simulink model "Q_learning_rotor_v3_min_M_imp"  (R2021a)
settings: Solver=VariableStepAuto  StartTime=0.0  StopTime=Tf  RelTol=1e-3
values from neighbouring files (symbols this model uses):
  Ator = pi*r^2    (= 0.00125663706144)    [INIT_rotor.m]    (also in rotor_DataFile.m)
  bd = 20    [INIT_rotor.m]    (also in rotor_DataFile.m)
  deltam = 0    [INIT_rotor.m]    (also in rotor_DataFile.m = 3e-05)
  dumax = ustavka+0.2e-3    (= 0.0034)    [INIT_Q_rotor.m]
  dumin = ustavka-0.2e-3    (= 0.003)    [INIT_Q_rotor.m]
  kd = 8e3    (= 8000)    [INIT_rotor.m]    (also in rotor_DataFile.m)
  Kr = 1000    [INIT_Q_rotor.m]
  n = -3e+3    (= -3000)    [INIT_rotor.m]    (also in rotor_DataFile.m)
  p0 = 1.08e5    (= 108000)    [rotor_DataFile.m]
  p00 = 1.05e5    (= 105000)    [rotor_DataFile.m]
  p0max = 1.1e5    (= 110000)    [INIT_Q_rotor.m]
  p0min = 1.05e5    (= 105000)    [INIT_Q_rotor.m]
  p1 = 1.08e5    (= 108000)    [rotor_DataFile.m]
  p10 = 1.00e5    (= 100000)    [rotor_DataFile.m]
  p11 = 1.00e5    (= 100000)    [INIT_rotor.m]
  p1max = 1.08e5    (= 108000)    [INIT_Q_rotor.m]
  p1min = 1e5    (= 100000)    [INIT_Q_rotor.m]
  Tf = 4    [INIT_Q_rotor.m]
  ustavka = 3.2e-3    (= 0.0032)    [INIT_Q_rotor.m]
  X10 = 1    [INIT_rotor.m]    (also in rotor_DataFile.m = 0)
  X20 = 0    [INIT_rotor.m]    (also in rotor_DataFile.m)
  X30 = 200    [INIT_rotor.m]
undefined symbols (not defined in the file or in its folder): smiData, X, Y, Z
libraries: neural x80, sm_lib x21, nesl_utility x14, simulink x7, dspmathops x3, pid_lib x1, rllib x1
(part 4 of 4)

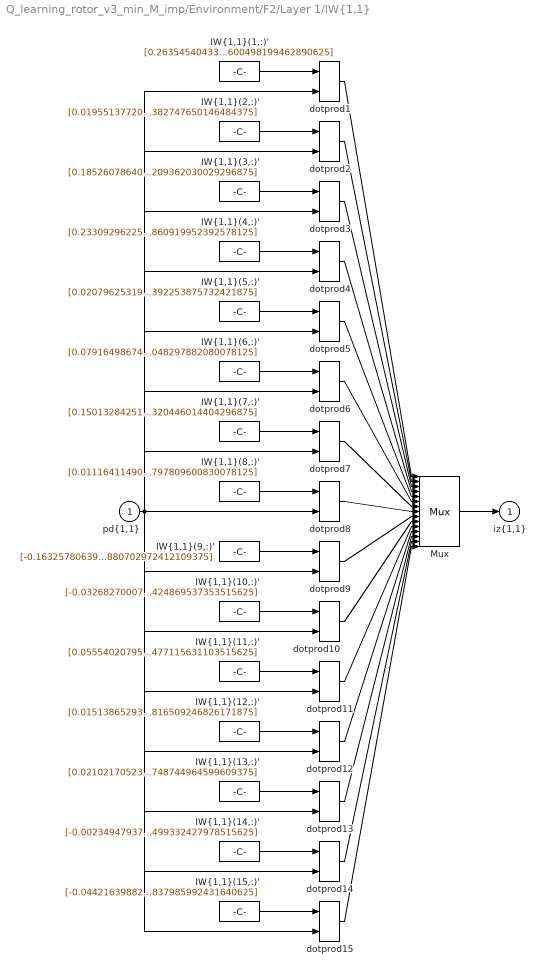
== system Q_learning_rotor_v3_min_M_imp/Environment/F2/Layer 1/IW{1,1} ==
  "pd{1,1}" : Inport  PortDimensions=8
      mask Display: e = 0.06;c1 = [120 230 180]/255;c2 = ([120 230 180]+0)/(256+128);c3 = ([120 230 180]+128)/(256+128);patch([0 1 1 0],[0 0 1 1],c1);patch([0 1 1 1-e 1-e 0+e],[0 0 1 1-e 0+e 0+e],c2);patch([0 0 1 1-e 0+e 0+e],[0 1 1 1-e 1-e 0+e],c3);plot([0 1 1 0 0],[0 0 1 1 0]);
  "IW{1,1}(1,:)'" : Constant  Value=[0.263545404332929056323564509511925280094146728515625;0.0280744574899199593465137780867735273204743862152099609375;0.785332970886842840485542183159850537776947021484375;-2.400750927396896106102985868346877396106719970703125;-1.03350617396331045938495662994682788848876953125;-1.2258655255748223122935769424657337367534637451171875;0.1567087824745667379300329002944636158645153045654296875;0.1216734266486191595735277815037989057600498199462890625]
      mask Display: e = 0.06;c1 = [120 150 230]/255;c2 = ([120 150 230]+0)/383;c3 = ([120 150 230]+128)/383;patch([0 1 1 0],[0 0 1 1],c1);patch([0 1 1 1-e 1-e 0+e],[0 0 1 1-e 0+e 0+e],c2);patch([0 0 1 1-e 0+e 0+e],[0 1 1 1-e 1-e 0+e],c3);plot([0 1 1 0 0],[0 0 1 1 0]);disp('Weights');
  "IW{1,1}(10,:)'" : Constant  Value=[-0.032682700078258054843249880150324315764009952545166015625;0.03781420832800962139597089617382152937352657318115234375;-1.3144429617808779386933792920899577438831329345703125;-2.681476711076717034387684179819189012050628662109375;-1.9744435884615196830083050372195430099964141845703125;0.94119793184532640761830180053948424756526947021484375;-1.019077215252574664106077761971391737461090087890625;0.0192143505873720345233923723071711719967424869537353515625]
      mask Display: e = 0.06;c1 = [120 150 230]/255;c2 = ([120 150 230]+0)/383;c3 = ([120 150 230]+128)/383;patch([0 1 1 0],[0 0 1 1],c1);patch([0 1 1 1-e 1-e 0+e],[0 0 1 1-e 0+e 0+e],c2);patch([0 0 1 1-e 0+e 0+e],[0 1 1 1-e 1-e 0+e],c3);plot([0 1 1 0 0],[0 0 1 1 0]);disp('Weights');
  "IW{1,1}(11,:)'" : Constant  Value=[0.055540207952238344890627530503479647450149059295654296875;0.00866395649697577173442564202332505374215543270111083984375;-0.1495569984123192586178419105635839514434337615966796875;-1.2041741748349570340081982067204080522060394287109375;-0.56109907977361472841693057489464990794658660888671875;-0.367585963305995855332497512790723703801631927490234375;-0.4099183908587580305038500227965414524078369140625;0.032207486974964817660893601214411319233477115631103515625]
      mask Display: e = 0.06;c1 = [120 150 230]/255;c2 = ([120 150 230]+0)/383;c3 = ([120 150 230]+128)/383;patch([0 1 1 0],[0 0 1 1],c1);patch([0 1 1 1-e 1-e 0+e],[0 0 1 1-e 0+e 0+e],c2);patch([0 0 1 1-e 0+e 0+e],[0 1 1 1-e 1-e 0+e],c3);plot([0 1 1 0 0],[0 0 1 1 0]);disp('Weights');
  "IW{1,1}(12,:)'" : Constant  Value=[0.01513865293832539204998965942650102078914642333984375;-0.007286743139548861221410636090922707808203995227813720703125;0.08408901881263618205419874129802337847650051116943359375;0.14107413188811068760486477913218550384044647216796875;1.2293671603681011195163819138542748987674713134765625;0.405997235974045300732626628814614377915859222412109375;-0.93506324769651960604477380911703221499919891357421875;-0.00684806045102126330348379923407264868728816509246826171875]
      mask Display: e = 0.06;c1 = [120 150 230]/255;c2 = ([120 150 230]+0)/383;c3 = ([120 150 230]+128)/383;patch([0 1 1 0],[0 0 1 1],c1);patch([0 1 1 1-e 1-e 0+e],[0 0 1 1-e 0+e 0+e],c2);patch([0 0 1 1-e 0+e 0+e],[0 1 1 1-e 1-e 0+e],c3);plot([0 1 1 0 0],[0 0 1 1 0]);disp('Weights');
  "IW{1,1}(13,:)'" : Constant  Value=[0.0210217052303556528602968000996042974293231964111328125;-0.032273386069569386103150776534675969742238521575927734375;0.1523531376308588647372488367182086221873760223388671875;-0.50578406248212903761896086507476866245269775390625;-1.2148553203552625578964807573356665670871734619140625;0.93089507593940756802197711294866167008876800537109375;0.8797008886075923239644680506899021565914154052734375;-0.01011072435612333196564005532991359359584748744964599609375]
      mask Display: e = 0.06;c1 = [120 150 230]/255;c2 = ([120 150 230]+0)/383;c3 = ([120 150 230]+128)/383;patch([0 1 1 0],[0 0 1 1],c1);patch([0 1 1 1-e 1-e 0+e],[0 0 1 1-e 0+e 0+e],c2);patch([0 0 1 1-e 0+e 0+e],[0 1 1 1-e 1-e 0+e],c3);plot([0 1 1 0 0],[0 0 1 1 0]);disp('Weights');
  "IW{1,1}(14,:)'" : Constant  Value=[-0.002349479374296047085035610280101536773145198822021484375;-0.015503507698309160200977885324391536414623260498046875;-0.393141378679239650306698194981436245143413543701171875;0.10230100857625297472441872059789602644741535186767578125;-0.0985401080283706265472432050955831073224544525146484375;0.256601592956030966075076094057294540107250213623046875;-0.69141570456732670546529107014066539704799652099609375;0.061357359811551694106501741998727084137499332427978515625]
      mask Display: e = 0.06;c1 = [120 150 230]/255;c2 = ([120 150 230]+0)/383;c3 = ([120 150 230]+128)/383;patch([0 1 1 0],[0 0 1 1],c1);patch([0 1 1 1-e 1-e 0+e],[0 0 1 1-e 0+e 0+e],c2);patch([0 0 1 1-e 0+e 0+e],[0 1 1 1-e 1-e 0+e],c3);plot([0 1 1 0 0],[0 0 1 1 0]);disp('Weights');
  "IW{1,1}(15,:)'" : Constant  Value=[-0.044216398821182827105769064246487687341868877410888671875;0.0150412139294658873944765531405209912918508052825927734375;-0.56415725694198382011990133833023719489574432373046875;1.5027241430763869090014850371517241001129150390625;0.355737529627508541896219185218797065317630767822265625;0.67099091817371192547625469160266220569610595703125;0.864116878011450761931655506487004458904266357421875;-0.07105011406486406999594152011923142708837985992431640625]
      mask Display: e = 0.06;c1 = [120 150 230]/255;c2 = ([120 150 230]+0)/383;c3 = ([120 150 230]+128)/383;patch([0 1 1 0],[0 0 1 1],c1);patch([0 1 1 1-e 1-e 0+e],[0 0 1 1-e 0+e 0+e],c2);patch([0 0 1 1-e 0+e 0+e],[0 1 1 1-e 1-e 0+e],c3);plot([0 1 1 0 0],[0 0 1 1 0]);disp('Weights');
  "IW{1,1}(2,:)'" : Constant  Value=[0.0195513772009782982319592292697052471339702606201171875;-0.01018554910181642715605310200999156222678720951080322265625;1.0376137849348501251967036296264268457889556884765625;0.403408290930529156437245319466455839574337005615234375;-0.665510220609730307472773347399197518825531005859375;-0.51058035967489578954570106361643411219120025634765625;1.0007272117893375451558313216082751750946044921875;0.019596135259655055038674476008964120410382747650146484375]
      mask Display: e = 0.06;c1 = [120 150 230]/255;c2 = ([120 150 230]+0)/383;c3 = ([120 150 230]+128)/383;patch([0 1 1 0],[0 0 1 1],c1);patch([0 1 1 1-e 1-e 0+e],[0 0 1 1-e 0+e 0+e],c2);patch([0 0 1 1-e 0+e 0+e],[0 1 1 1-e 1-e 0+e],c3);plot([0 1 1 0 0],[0 0 1 1 0]);disp('Weights');
  "IW{1,1}(3,:)'" : Constant  Value=[0.1852607864006721449801062817641650326550006866455078125;-0.035421893108780903858257005367704550735652446746826171875;-0.96238883016556642235883600733359344303607940673828125;-0.1398795408219530578275424659295822493731975555419921875;0.043315733871104648844418960607072222046554088592529296875;0.74905077928134866649401146787567995488643646240234375;-1.3480146194933546599514784247730858623981475830078125;0.158637073539034278990556003918754868209362030029296875]
      mask Display: e = 0.06;c1 = [120 150 230]/255;c2 = ([120 150 230]+0)/383;c3 = ([120 150 230]+128)/383;patch([0 1 1 0],[0 0 1 1],c1);patch([0 1 1 1-e 1-e 0+e],[0 0 1 1-e 0+e 0+e],c2);patch([0 0 1 1-e 0+e 0+e],[0 1 1 1-e 1-e 0+e],c3);plot([0 1 1 0 0],[0 0 1 1 0]);disp('Weights');
  "IW{1,1}(4,:)'" : Constant  Value=[0.23309296225073039554587239763350225985050201416015625;0.03210029035712336220598217551014386117458343505859375;0.65784775936412243080297912456444464623928070068359375;-2.453647203103570095805707751424051821231842041015625;-1.1857418175884053557211927909520454704761505126953125;-1.0833997280227725124035487169749103486537933349609375;0.053272902877193495374541498676990158855915069580078125;0.12026706771248170391164222792212967760860919952392578125]
      mask Display: e = 0.06;c1 = [120 150 230]/255;c2 = ([120 150 230]+0)/383;c3 = ([120 150 230]+128)/383;patch([0 1 1 0],[0 0 1 1],c1);patch([0 1 1 1-e 1-e 0+e],[0 0 1 1-e 0+e 0+e],c2);patch([0 0 1 1-e 0+e 0+e],[0 1 1 1-e 1-e 0+e],c3);plot([0 1 1 0 0],[0 0 1 1 0]);disp('Weights');
  "IW{1,1}(5,:)'" : Constant  Value=[0.0207962531983513047861844569297318230383098125457763671875;0.0258380085905217903030628434635218582116067409515380859375;-0.75225209845463492097650259893271140754222869873046875;-1.8055881558413087173420308317872695624828338623046875;-1.2661925975772041486067109872237779200077056884765625;0.30820038911983738127986498511745594441890716552734375;-0.69762588488066878955606853196513839066028594970703125;0.043450823381268655065667871895129792392253875732421875]
      mask Display: e = 0.06;c1 = [120 150 230]/255;c2 = ([120 150 230]+0)/383;c3 = ([120 150 230]+128)/383;patch([0 1 1 0],[0 0 1 1],c1);patch([0 1 1 1-e 1-e 0+e],[0 0 1 1-e 0+e 0+e],c2);patch([0 0 1 1-e 0+e 0+e],[0 1 1 1-e 1-e 0+e],c3);plot([0 1 1 0 0],[0 0 1 1 0]);disp('Weights');
  "IW{1,1}(6,:)'" : Constant  Value=[0.0791649867434642551256018805361236445605754852294921875;-0.0208260864341522251852456548704140004701912403106689453125;-0.541038515794388441548790069646202027797698974609375;0.01404869201285276723856210168150937533937394618988037109375;-0.05333402617709774584664472740769269876182079315185546875;0.4645797256487174120564986878889612853527069091796875;-0.86253689600163496731255463600973598659038543701171875;0.08261879415788993263891626384065602906048297882080078125]
      mask Display: e = 0.06;c1 = [120 150 230]/255;c2 = ([120 150 230]+0)/383;c3 = ([120 150 230]+128)/383;patch([0 1 1 0],[0 0 1 1],c1);patch([0 1 1 1-e 1-e 0+e],[0 0 1 1-e 0+e 0+e],c2);patch([0 0 1 1-e 0+e 0+e],[0 1 1 1-e 1-e 0+e],c3);plot([0 1 1 0 0],[0 0 1 1 0]);disp('Weights');
  "IW{1,1}(7,:)'" : Constant  Value=[0.1501328425117599840721283044331357814371585845947265625;-0.1419145374554392213806153222321881912648677825927734375;-0.50031355222014750605552535489550791680812835693359375;1.0439359379314641085301218481617979705333709716796875;0.2296139652304131362203776234309771098196506500244140625;-0.768687381273901682021687520318664610385894775390625;0.327858303858620081516761501916334964334964752197265625;-0.5721788946593224789438636435079388320446014404296875]
      mask Display: e = 0.06;c1 = [120 150 230]/255;c2 = ([120 150 230]+0)/383;c3 = ([120 150 230]+128)/383;patch([0 1 1 0],[0 0 1 1],c1);patch([0 1 1 1-e 1-e 0+e],[0 0 1 1-e 0+e 0+e],c2);patch([0 0 1 1-e 0+e 0+e],[0 1 1 1-e 1-e 0+e],c3);plot([0 1 1 0 0],[0 0 1 1 0]);disp('Weights');
  "IW{1,1}(8,:)'" : Constant  Value=[0.0111641149092882967230888624499129946343600749969482421875;0.019322299447494285795645652115126722492277622222900390625;0.6476794046053793163508771613123826682567596435546875;-1.9590535910084947435194635545485652983188629150390625;-0.95194517339799744615191912089358083903789520263671875;-0.2051910504571095306136641056582448072731494903564453125;-0.34028428786666464755938932285062037408351898193359375;0.1531810528174038232851472685069893486797809600830078125]
      mask Display: e = 0.06;c1 = [120 150 230]/255;c2 = ([120 150 230]+0)/383;c3 = ([120 150 230]+128)/383;patch([0 1 1 0],[0 0 1 1],c1);patch([0 1 1 1-e 1-e 0+e],[0 0 1 1-e 0+e 0+e],c2);patch([0 0 1 1-e 0+e 0+e],[0 1 1 1-e 1-e 0+e],c3);plot([0 1 1 0 0],[0 0 1 1 0]);disp('Weights');
  "IW{1,1}(9,:)'" : Constant  Value=[-0.1632578063934266576762155409596743993461132049560546875;0.049121285080663816546842070920320111326873302459716796875;0.70710307107203906884507205177214927971363067626953125;0.74083810589253185074909424656652845442295074462890625;-0.79287321140284994225311265836353413760662078857421875;0.6505880433479329649770761534455232322216033935546875;0.86903557929343555610302018976653926074504852294921875;-0.17748956420124917254810270605958066880702972412109375]
      mask Display: e = 0.06;c1 = [120 150 230]/255;c2 = ([120 150 230]+0)/383;c3 = ([120 150 230]+128)/383;patch([0 1 1 0],[0 0 1 1],c1);patch([0 1 1 1-e 1-e 0+e],[0 0 1 1-e 0+e 0+e],c2);patch([0 0 1 1-e 0+e 0+e],[0 1 1 1-e 1-e 0+e],c3);plot([0 1 1 0 0],[0 0 1 1 0]);disp('Weights');
  Mux : Mux  Inputs=15
      mask Display: e = 0.06;c1 = [120 150 230]/255;c2 = ([120 150 230]+0)/383;c3 = ([120 150 230]+128)/383;patch([0 1 1 0],[0 0 1 1],c1);patch([0 1 1 1-e 1-e 0+e],[0 0 1 1-e 0+e 0+e],c2);patch([0 0 1 1-e 0+e 0+e],[0 1 1 1-e 1-e 0+e],c3);plot([0 1 1 0 0],[0 0 1 1 0]);disp('Mux');
  dotprod{1..15} (15 alike) : neural/Weight Functions/dotprod
  "iz{1,1}" : Outport
      mask Display: e = 0.06;c1 = [120 230 180]/255;c2 = ([120 230 180]+0)/(256+128);c3 = ([120 230 180]+128)/(256+128);patch([0 1 1 0],[0 0 1 1],c1);patch([0 1 1 1-e 1-e 0+e],[0 0 1 1-e 0+e 0+e],c2);patch([0 0 1 1-e 0+e 0+e],[0 1 1 1-e 1-e 0+e],c3);plot([0 1 1 0 0],[0 0 1 1 0]);
  wires:
  "IW{1,1}(1,:)'"/1 -> dotprod1/1
  "pd{1,1}"/1 -> dotprod1/2, dotprod2/2, dotprod3/2, dotprod4/2, dotprod5/2, dotprod6/2, dotprod7/2, dotprod8/2, dotprod9/2, dotprod10/2, dotprod11/2, dotprod12/2, dotprod13/2, dotprod14/2, dotprod15/2
  dotprod1/1 -> Mux/1
  "IW{1,1}(2,:)'"/1 -> dotprod2/1
  dotprod2/1 -> Mux/2
  "IW{1,1}(3,:)'"/1 -> dotprod3/1
  dotprod3/1 -> Mux/3
  "IW{1,1}(4,:)'"/1 -> dotprod4/1
  dotprod4/1 -> Mux/4
  "IW{1,1}(5,:)'"/1 -> dotprod5/1
  dotprod5/1 -> Mux/5
  "IW{1,1}(6,:)'"/1 -> dotprod6/1
  dotprod6/1 -> Mux/6
  "IW{1,1}(7,:)'"/1 -> dotprod7/1
  dotprod7/1 -> Mux/7
  "IW{1,1}(8,:)'"/1 -> dotprod8/1
  dotprod8/1 -> Mux/8
  "IW{1,1}(9,:)'"/1 -> dotprod9/1
  dotprod9/1 -> Mux/9
  "IW{1,1}(10,:)'"/1 -> dotprod10/1
  dotprod10/1 -> Mux/10
  "IW{1,1}(11,:)'"/1 -> dotprod11/1
  dotprod11/1 -> Mux/11
  "IW{1,1}(12,:)'"/1 -> dotprod12/1
  dotprod12/1 -> Mux/12
  "IW{1,1}(13,:)'"/1 -> dotprod13/1
  dotprod13/1 -> Mux/13
  "IW{1,1}(14,:)'"/1 -> dotprod14/1
  dotprod14/1 -> Mux/14
  "IW{1,1}(15,:)'"/1 -> dotprod15/1
  dotprod15/1 -> Mux/15
  Mux/1 -> "iz{1,1}"/1

== system Q_learning_rotor_v3_min_M_imp/Environment/F2/Layer 2/Delays 1 ==
  "p{2}" : Inport  PortDimensions=15
      mask Display: e = 0.06;c1 = [120 230 180]/255;c2 = ([120 230 180]+0)/(256+128);c3 = ([120 230 180]+128)/(256+128);patch([0 1 1 0],[0 0 1 1],c1);patch([0 1 1 1-e 1-e 0+e],[0 0 1 1-e 0+e 0+e],c2);patch([0 0 1 1-e 0+e 0+e],[0 1 1 1-e 1-e 0+e],c3);plot([0 1 1 0 0],[0 0 1 1 0]);
  mux : Mux  Inputs=1
      mask Display: e = 0.06;c1 = [120 150 230]/255;c2 = ([120 150 230]+0)/383;c3 = ([120 150 230]+128)/383;patch([0 1 1 0],[0 0 1 1],c1);patch([0 1 1 1-e 1-e 0+e],[0 0 1 1-e 0+e 0+e],c2);patch([0 0 1 1-e 0+e 0+e],[0 1 1 1-e 1-e 0+e],c3);plot([0 1 1 0 0],[0 0 1 1 0]);disp('Mux')
  "pd{2,1}" : Outport
      mask Display: e = 0.06;c1 = [120 230 180]/255;c2 = ([120 230 180]+0)/(256+128);c3 = ([120 230 180]+128)/(256+128);patch([0 1 1 0],[0 0 1 1],c1);patch([0 1 1 1-e 1-e 0+e],[0 0 1 1-e 0+e 0+e],c2);patch([0 0 1 1-e 0+e 0+e],[0 1 1 1-e 1-e 0+e],c3);plot([0 1 1 0 0],[0 0 1 1 0]);
  wires:
  "p{2}"/1 -> mux/1
  mux/1 -> "pd{2,1}"/1

== system Q_learning_rotor_v3_min_M_imp/Environment/F2/Layer 2/LW{2,1} ==
  "ad{2,1}" : Inport  PortDimensions=15
      mask Display: e = 0.06;c1 = [120 230 180]/255;c2 = ([120 230 180]+0)/(256+128);c3 = ([120 230 180]+128)/(256+128);patch([0 1 1 0],[0 0 1 1],c1);patch([0 1 1 1-e 1-e 0+e],[0 0 1 1-e 0+e 0+e],c2);patch([0 0 1 1-e 0+e 0+e],[0 1 1 1-e 1-e 0+e],c3);plot([0 1 1 0 0],[0 0 1 1 0]);
  "IW{2,1}(1,:)'" : Constant  Value=[-2.8839445060521295971511790412478148937225341796875;7.68490157682992514054376442800275981426239013671875;1.6083510919674959271929992610239423811435699462890625;3.49943182265510532857888392754830420017242431640625;-3.8525253166788360204009222798049449920654296875;-5.88610951123064385370753370807506144046783447265625;0.033877648943551226523585029326568474061787128448486328125;-3.281568649392260450525782289332710206508636474609375;0.2124320347898714100853823083525639958679676055908203125;1.26767619245783347281530950567685067653656005859375;1.6439680904654132564957080830936320126056671142578125;-3.4066905868457890704803503467701375484466552734375;-9.6163191123424436312916441238485276699066162109375;4.4120135957978714458249669405631721019744873046875;-4.388737037437319798982571228407323360443115234375]
      mask Display: e = 0.06;c1 = [120 150 230]/255;c2 = ([120 150 230]+0)/383;c3 = ([120 150 230]+128)/383;patch([0 1 1 0],[0 0 1 1],c1);patch([0 1 1 1-e 1-e 0+e],[0 0 1 1-e 0+e 0+e],c2);patch([0 0 1 1-e 0+e 0+e],[0 1 1 1-e 1-e 0+e],c3);plot([0 1 1 0 0],[0 0 1 1 0]);disp('weights');
  Mux : Mux  Inputs=1
      mask Display: e = 0.06;c1 = [120 150 230]/255;c2 = ([120 150 230]+0)/383;c3 = ([120 150 230]+128)/383;patch([0 1 1 0],[0 0 1 1],c1);patch([0 1 1 1-e 1-e 0+e],[0 0 1 1-e 0+e 0+e],c2);patch([0 0 1 1-e 0+e 0+e],[0 1 1 1-e 1-e 0+e],c3);plot([0 1 1 0 0],[0 0 1 1 0]);disp('Mux');
  dotprod1 : neural/Weight Functions/dotprod
  "lz{2,1}" : Outport
      mask Display: e = 0.06;c1 = [120 230 180]/255;c2 = ([120 230 180]+0)/(256+128);c3 = ([120 230 180]+128)/(256+128);patch([0 1 1 0],[0 0 1 1],c1);patch([0 1 1 1-e 1-e 0+e],[0 0 1 1-e 0+e 0+e],c2);patch([0 0 1 1-e 0+e 0+e],[0 1 1 1-e 1-e 0+e],c3);plot([0 1 1 0 0],[0 0 1 1 0]);
  wires:
  "IW{2,1}(1,:)'"/1 -> dotprod1/1
  "ad{2,1}"/1 -> dotprod1/2
  dotprod1/1 -> Mux/1
  Mux/1 -> "lz{2,1}"/1

== system Q_learning_rotor_v3_min_M_imp/Environment/F3/Layer 1/Delays 1 ==
  "p{1}" : Inport  PortDimensions=8
      mask Display: e = 0.06;c1 = [120 230 180]/255;c2 = ([120 230 180]+0)/(256+128);c3 = ([120 230 180]+128)/(256+128);patch([0 1 1 0],[0 0 1 1],c1);patch([0 1 1 1-e 1-e 0+e],[0 0 1 1-e 0+e 0+e],c2);patch([0 0 1 1-e 0+e 0+e],[0 1 1 1-e 1-e 0+e],c3);plot([0 1 1 0 0],[0 0 1 1 0]);
  mux : Mux  Inputs=1
      mask Display: e = 0.06;c1 = [120 150 230]/255;c2 = ([120 150 230]+0)/383;c3 = ([120 150 230]+128)/383;patch([0 1 1 0],[0 0 1 1],c1);patch([0 1 1 1-e 1-e 0+e],[0 0 1 1-e 0+e 0+e],c2);patch([0 0 1 1-e 0+e 0+e],[0 1 1 1-e 1-e 0+e],c3);plot([0 1 1 0 0],[0 0 1 1 0]);disp('Mux')
  "pd{1,1}" : Outport
      mask Display: e = 0.06;c1 = [120 230 180]/255;c2 = ([120 230 180]+0)/(256+128);c3 = ([120 230 180]+128)/(256+128);patch([0 1 1 0],[0 0 1 1],c1);patch([0 1 1 1-e 1-e 0+e],[0 0 1 1-e 0+e 0+e],c2);patch([0 0 1 1-e 0+e 0+e],[0 1 1 1-e 1-e 0+e],c3);plot([0 1 1 0 0],[0 0 1 1 0]);
  wires:
  "p{1}"/1 -> mux/1
  mux/1 -> "pd{1,1}"/1

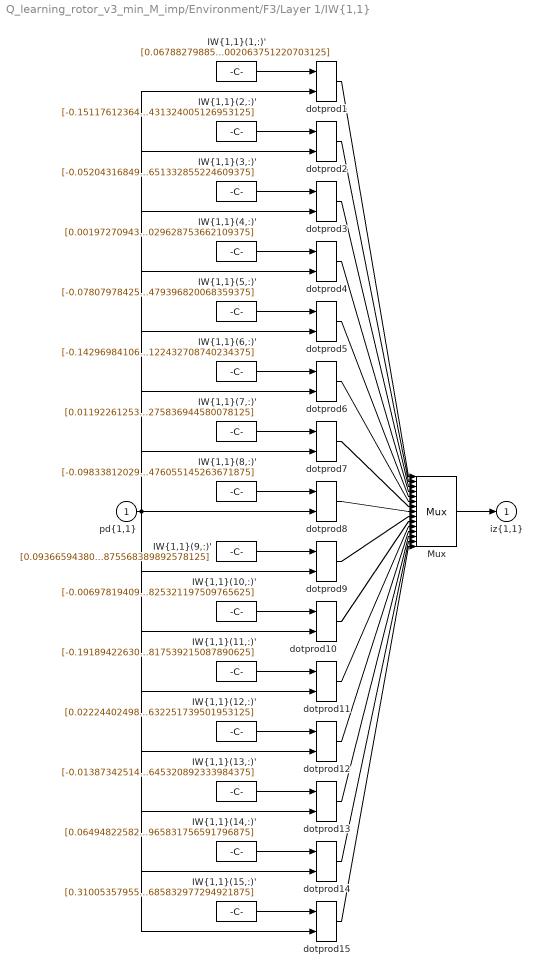
== system Q_learning_rotor_v3_min_M_imp/Environment/F3/Layer 1/IW{1,1} ==
  "pd{1,1}" : Inport  PortDimensions=8
      mask Display: e = 0.06;c1 = [120 230 180]/255;c2 = ([120 230 180]+0)/(256+128);c3 = ([120 230 180]+128)/(256+128);patch([0 1 1 0],[0 0 1 1],c1);patch([0 1 1 1-e 1-e 0+e],[0 0 1 1-e 0+e 0+e],c2);patch([0 0 1 1-e 0+e 0+e],[0 1 1 1-e 1-e 0+e],c3);plot([0 1 1 0 0],[0 0 1 1 0]);
  "IW{1,1}(1,:)'" : Constant  Value=[0.06788279885655380818665349806906306184828281402587890625;-0.00992236614156143115206276661410811357200145721435546875;0.128807470069277008040131704547093249857425689697265625;-2.07557374820626261424649783293716609477996826171875;-1.3371842639701483346215127312461845576763153076171875;-2.173773926338138817726530760410241782665252685546875;-0.854299781709458638800924745737574994564056396484375;0.06477886523293803489043085619414341636002063751220703125]
      mask Display: e = 0.06;c1 = [120 150 230]/255;c2 = ([120 150 230]+0)/383;c3 = ([120 150 230]+128)/383;patch([0 1 1 0],[0 0 1 1],c1);patch([0 1 1 1-e 1-e 0+e],[0 0 1 1-e 0+e 0+e],c2);patch([0 0 1 1-e 0+e 0+e],[0 1 1 1-e 1-e 0+e],c3);plot([0 1 1 0 0],[0 0 1 1 0]);disp('Weights');
  "IW{1,1}(10,:)'" : Constant  Value=[-0.006978194095090421711358175116401980631053447723388671875;0.00922221332153015660448858170639141462743282318115234375;-0.330894108761513872085657794741564430296421051025390625;0.8886342899794936744939377604168839752674102783203125;-0.351152275670796931716921562838251702487468719482421875;0.9474812931835525642298989623668603599071502685546875;1.021305796765827000882609354448504745960235595703125;-0.037725419671657024756061815651264623738825321197509765625]
      mask Display: e = 0.06;c1 = [120 150 230]/255;c2 = ([120 150 230]+0)/383;c3 = ([120 150 230]+128)/383;patch([0 1 1 0],[0 0 1 1],c1);patch([0 1 1 1-e 1-e 0+e],[0 0 1 1-e 0+e 0+e],c2);patch([0 0 1 1-e 0+e 0+e],[0 1 1 1-e 1-e 0+e],c3);plot([0 1 1 0 0],[0 0 1 1 0]);disp('Weights');
  "IW{1,1}(11,:)'" : Constant  Value=[-0.1918942263094554900870747360386303626000881195068359375;-0.0045254450572274999842203868638534913770854473114013671875;0.898112362451640944271957778255455195903778076171875;0.216610886716492812009704493902972899377346038818359375;-0.5903638625466645084571837287512607872486114501953125;-2.03988383709788489994707560981623828411102294921875;0.133448489177298179608754935543402098119258880615234375;0.149400957588209204462970092208706773817539215087890625]
      mask Display: e = 0.06;c1 = [120 150 230]/255;c2 = ([120 150 230]+0)/383;c3 = ([120 150 230]+128)/383;patch([0 1 1 0],[0 0 1 1],c1);patch([0 1 1 1-e 1-e 0+e],[0 0 1 1-e 0+e 0+e],c2);patch([0 0 1 1-e 0+e 0+e],[0 1 1 1-e 1-e 0+e],c3);plot([0 1 1 0 0],[0 0 1 1 0]);disp('Weights');
  "IW{1,1}(12,:)'" : Constant  Value=[0.0222440249845849737087011277480996795929968357086181640625;0.00650835675493242372946500751140774809755384922027587890625;0.2126146796901738633689404878168716095387935638427734375;0.22473885325326126150002892245538532733917236328125;-0.77026826774832157784800301669747568666934967041015625;-0.42125467116819759194612515784683637320995330810546875;0.83276323841456501018143399051041342318058013916015625;0.017557852814675374564234999752443400211632251739501953125]
      mask Display: e = 0.06;c1 = [120 150 230]/255;c2 = ([120 150 230]+0)/383;c3 = ([120 150 230]+128)/383;patch([0 1 1 0],[0 0 1 1],c1);patch([0 1 1 1-e 1-e 0+e],[0 0 1 1-e 0+e 0+e],c2);patch([0 0 1 1-e 0+e 0+e],[0 1 1 1-e 1-e 0+e],c3);plot([0 1 1 0 0],[0 0 1 1 0]);disp('Weights');
  "IW{1,1}(13,:)'" : Constant  Value=[-0.01387342514656162047181897634118286077864468097686767578125;0.01297421504082907350863251849659718573093414306640625;-0.631599189159698592987979282042942941188812255859375;-0.9796428852581460233750476618297398090362548828125;-0.0383016700428938372535725420675589703023433685302734375;-1.6157790195434416080644268731703050434589385986328125;-1.0822132089536109500471638966700993478298187255859375;0.052192302752546236577213534246766357682645320892333984375]
      mask Display: e = 0.06;c1 = [120 150 230]/255;c2 = ([120 150 230]+0)/383;c3 = ([120 150 230]+128)/383;patch([0 1 1 0],[0 0 1 1],c1);patch([0 1 1 1-e 1-e 0+e],[0 0 1 1-e 0+e 0+e],c2);patch([0 0 1 1-e 0+e 0+e],[0 1 1 1-e 1-e 0+e],c3);plot([0 1 1 0 0],[0 0 1 1 0]);disp('Weights');
  "IW{1,1}(14,:)'" : Constant  Value=[0.06494822582515873132802397549312445335090160369873046875;0.01179147852846387616032597378534774179570376873016357421875;-0.55416769562306011920327364350669085979461669921875;-0.7851185296991458617554826560080982744693756103515625;-0.353385480256569295409718733935733325779438018798828125;1.9326126031133357141555961788981221616268157958984375;0.318004305208750615019397400828893296420574188232421875;-0.041408834171954171654572718352937954477965831756591796875]
      mask Display: e = 0.06;c1 = [120 150 230]/255;c2 = ([120 150 230]+0)/383;c3 = ([120 150 230]+128)/383;patch([0 1 1 0],[0 0 1 1],c1);patch([0 1 1 1-e 1-e 0+e],[0 0 1 1-e 0+e 0+e],c2);patch([0 0 1 1-e 0+e 0+e],[0 1 1 1-e 1-e 0+e],c3);plot([0 1 1 0 0],[0 0 1 1 0]);disp('Weights');
  "IW{1,1}(15,:)'" : Constant  Value=[0.310053579551866909103097214028821326792240142822265625;-0.003967058471211982496884562721106703975237905979156494140625;-1.1384331891469832154228924991912208497524261474609375;-0.1774212528405465227887560786257381550967693328857421875;1.0456562539913416554071545760962180793285369873046875;2.177732673321708833924503778689540922641754150390625;-0.436451307036899549540720499862800352275371551513671875;-0.2422999450589031489311508948958362452685832977294921875]
      mask Display: e = 0.06;c1 = [120 150 230]/255;c2 = ([120 150 230]+0)/383;c3 = ([120 150 230]+128)/383;patch([0 1 1 0],[0 0 1 1],c1);patch([0 1 1 1-e 1-e 0+e],[0 0 1 1-e 0+e 0+e],c2);patch([0 0 1 1-e 0+e 0+e],[0 1 1 1-e 1-e 0+e],c3);plot([0 1 1 0 0],[0 0 1 1 0]);disp('Weights');
  "IW{1,1}(2,:)'" : Constant  Value=[-0.1511761236496747262680884205110487528145313262939453125;-0.00881789659697155940587531830487932893447577953338623046875;-0.1261543085943037656448950656340457499027252197265625;0.489396239657587217575240856604068540036678314208984375;-0.2207616966116522638774455344901070930063724517822265625;0.251424731887772423544191724431584589183330535888671875;0.097557007687249230887260864619747735559940338134765625;0.0239275744022753762696442692003984120674431324005126953125]
      mask Display: e = 0.06;c1 = [120 150 230]/255;c2 = ([120 150 230]+0)/383;c3 = ([120 150 230]+128)/383;patch([0 1 1 0],[0 0 1 1],c1);patch([0 1 1 1-e 1-e 0+e],[0 0 1 1-e 0+e 0+e],c2);patch([0 0 1 1-e 0+e 0+e],[0 1 1 1-e 1-e 0+e],c3);plot([0 1 1 0 0],[0 0 1 1 0]);disp('Weights');
  "IW{1,1}(3,:)'" : Constant  Value=[-0.05204316849955237245239914045669138431549072265625;0.00142568734179253863401937163501997929415665566921234130859375;-1.860726472222154814772920872201211750507354736328125;-1.3699586386795095105384234557277522981166839599609375;-0.288754708460629838651101408686372451484203338623046875;0.43689781072489697333338654061662964522838592529296875;-1.3054144450678315525493644599919207394123077392578125;0.005906429554605130416433667051023803651332855224609375]
      mask Display: e = 0.06;c1 = [120 150 230]/255;c2 = ([120 150 230]+0)/383;c3 = ([120 150 230]+128)/383;patch([0 1 1 0],[0 0 1 1],c1);patch([0 1 1 1-e 1-e 0+e],[0 0 1 1-e 0+e 0+e],c2);patch([0 0 1 1-e 0+e 0+e],[0 1 1 1-e 1-e 0+e],c3);plot([0 1 1 0 0],[0 0 1 1 0]);disp('Weights');
  "IW{1,1}(4,:)'" : Constant  Value=[0.001972709436021187479060046143786166794598102569580078125;-0.007549715445535030988732927426099195145070552825927734375;-1.196959391696092556145458729588426649570465087890625;-0.65884191472665321054336118322680704295635223388671875;-0.1867951756140261154737203241893439553678035736083984375;0.431106399485792712855669606142328120768070220947265625;-0.581805685047673382115362983313389122486114501953125;0.056432614527383816172001473887576139532029628753662109375]
      mask Display: e = 0.06;c1 = [120 150 230]/255;c2 = ([120 150 230]+0)/383;c3 = ([120 150 230]+128)/383;patch([0 1 1 0],[0 0 1 1],c1);patch([0 1 1 1-e 1-e 0+e],[0 0 1 1-e 0+e 0+e],c2);patch([0 0 1 1-e 0+e 0+e],[0 1 1 1-e 1-e 0+e],c3);plot([0 1 1 0 0],[0 0 1 1 0]);disp('Weights');
  "IW{1,1}(5,:)'" : Constant  Value=[-0.07807978425676752320949702834695926867425441741943359375;-0.00677429953288709828240765631335307261906564235687255859375;-0.0664314126019382999999152161763049662113189697265625;-0.386955493755659352128617456401116214692592620849609375;-0.0960269927478801521569806709521799348294734954833984375;-0.01720314009759908724372934329949202947318553924560546875;0.057611214507576093135643446885296725668013095855712890625;-0.0248487489313878005814384408722617081366479396820068359375]
      mask Display: e = 0.06;c1 = [120 150 230]/255;c2 = ([120 150 230]+0)/383;c3 = ([120 150 230]+128)/383;patch([0 1 1 0],[0 0 1 1],c1);patch([0 1 1 1-e 1-e 0+e],[0 0 1 1-e 0+e 0+e],c2);patch([0 0 1 1-e 0+e 0+e],[0 1 1 1-e 1-e 0+e],c3);plot([0 1 1 0 0],[0 0 1 1 0]);disp('Weights');
  "IW{1,1}(6,:)'" : Constant  Value=[-0.1429698410676345232683814856500248424708843231201171875;0.06679343247472328826130905099489609710872173309326171875;0.78610319187799693185780824933317489922046661376953125;0.98970498789565641839516274558263830840587615966796875;0.85264808828135041363083246324094943702220916748046875;-1.9128706056098938592668901037541218101978302001953125;0.838971287901387086094473488628864288330078125;0.1026202929340290503912314079570933245122432708740234375]
      mask Display: e = 0.06;c1 = [120 150 230]/255;c2 = ([120 150 230]+0)/383;c3 = ([120 150 230]+128)/383;patch([0 1 1 0],[0 0 1 1],c1);patch([0 1 1 1-e 1-e 0+e],[0 0 1 1-e 0+e 0+e],c2);patch([0 0 1 1-e 0+e 0+e],[0 1 1 1-e 1-e 0+e],c3);plot([0 1 1 0 0],[0 0 1 1 0]);disp('Weights');
  "IW{1,1}(7,:)'" : Constant  Value=[0.01192261253205783265440853568861712119542062282562255859375;0.002953547315193994111937048074878475745208561420440673828125;0.80887583328624590439659414187190122902393341064453125;-0.1311186120981299441101697311751195229589939117431640625;0.1442848684722133623115070122366887517273426055908203125;-0.25060501965799419910041478942730464041233062744140625;0.407150347884929264541398197252419777214527130126953125;-0.08340267370550531744743949502662871964275836944580078125]
      mask Display: e = 0.06;c1 = [120 150 230]/255;c2 = ([120 150 230]+0)/383;c3 = ([120 150 230]+128)/383;patch([0 1 1 0],[0 0 1 1],c1);patch([0 1 1 1-e 1-e 0+e],[0 0 1 1-e 0+e 0+e],c2);patch([0 0 1 1-e 0+e 0+e],[0 1 1 1-e 1-e 0+e],c3);plot([0 1 1 0 0],[0 0 1 1 0]);disp('Weights');
  "IW{1,1}(8,:)'" : Constant  Value=[-0.0983381202998495351774721484616748057305812835693359375;-0.002896860992941151409507671843357456964440643787384033203125;0.1773862169213134831746714326072833500802516937255859375;0.7067698616238973219338959097512997686862945556640625;-0.239147493231804675328788789556710980832576751708984375;0.1555922986075080338697063098152284510433673858642578125;0.52311960761349907134132308783591724932193756103515625;0.0264900577877667901816050033403371344320476055145263671875]
      mask Display: e = 0.06;c1 = [120 150 230]/255;c2 = ([120 150 230]+0)/383;c3 = ([120 150 230]+128)/383;patch([0 1 1 0],[0 0 1 1],c1);patch([0 1 1 1-e 1-e 0+e],[0 0 1 1-e 0+e 0+e],c2);patch([0 0 1 1-e 0+e 0+e],[0 1 1 1-e 1-e 0+e],c3);plot([0 1 1 0 0],[0 0 1 1 0]);disp('Weights');
  "IW{1,1}(9,:)'" : Constant  Value=[0.09366594380494457083852211098928819410502910614013671875;-0.01440292874345421199333561190769614768214523792266845703125;-0.3520744791741849955002408023574389517307281494140625;-0.8998918382846816665932010437245480716228485107421875;0.374977485732819026953421825965051539242267608642578125;-0.131297970009684183967380022295401431620121002197265625;-0.957166522100834527009283192455768585205078125;-0.0689537204583486051934215765868430025875568389892578125]
      mask Display: e = 0.06;c1 = [120 150 230]/255;c2 = ([120 150 230]+0)/383;c3 = ([120 150 230]+128)/383;patch([0 1 1 0],[0 0 1 1],c1);patch([0 1 1 1-e 1-e 0+e],[0 0 1 1-e 0+e 0+e],c2);patch([0 0 1 1-e 0+e 0+e],[0 1 1 1-e 1-e 0+e],c3);plot([0 1 1 0 0],[0 0 1 1 0]);disp('Weights');
  Mux : Mux  Inputs=15
      mask Display: e = 0.06;c1 = [120 150 230]/255;c2 = ([120 150 230]+0)/383;c3 = ([120 150 230]+128)/383;patch([0 1 1 0],[0 0 1 1],c1);patch([0 1 1 1-e 1-e 0+e],[0 0 1 1-e 0+e 0+e],c2);patch([0 0 1 1-e 0+e 0+e],[0 1 1 1-e 1-e 0+e],c3);plot([0 1 1 0 0],[0 0 1 1 0]);disp('Mux');
  dotprod{1..15} (15 alike) : neural/Weight Functions/dotprod
  "iz{1,1}" : Outport
      mask Display: e = 0.06;c1 = [120 230 180]/255;c2 = ([120 230 180]+0)/(256+128);c3 = ([120 230 180]+128)/(256+128);patch([0 1 1 0],[0 0 1 1],c1);patch([0 1 1 1-e 1-e 0+e],[0 0 1 1-e 0+e 0+e],c2);patch([0 0 1 1-e 0+e 0+e],[0 1 1 1-e 1-e 0+e],c3);plot([0 1 1 0 0],[0 0 1 1 0]);
  wires:
  "IW{1,1}(1,:)'"/1 -> dotprod1/1
  "pd{1,1}"/1 -> dotprod1/2, dotprod2/2, dotprod3/2, dotprod4/2, dotprod5/2, dotprod6/2, dotprod7/2, dotprod8/2, dotprod9/2, dotprod10/2, dotprod11/2, dotprod12/2, dotprod13/2, dotprod14/2, dotprod15/2
  dotprod1/1 -> Mux/1
  "IW{1,1}(2,:)'"/1 -> dotprod2/1
  dotprod2/1 -> Mux/2
  "IW{1,1}(3,:)'"/1 -> dotprod3/1
  dotprod3/1 -> Mux/3
  "IW{1,1}(4,:)'"/1 -> dotprod4/1
  dotprod4/1 -> Mux/4
  "IW{1,1}(5,:)'"/1 -> dotprod5/1
  dotprod5/1 -> Mux/5
  "IW{1,1}(6,:)'"/1 -> dotprod6/1
  dotprod6/1 -> Mux/6
  "IW{1,1}(7,:)'"/1 -> dotprod7/1
  dotprod7/1 -> Mux/7
  "IW{1,1}(8,:)'"/1 -> dotprod8/1
  dotprod8/1 -> Mux/8
  "IW{1,1}(9,:)'"/1 -> dotprod9/1
  dotprod9/1 -> Mux/9
  "IW{1,1}(10,:)'"/1 -> dotprod10/1
  dotprod10/1 -> Mux/10
  "IW{1,1}(11,:)'"/1 -> dotprod11/1
  dotprod11/1 -> Mux/11
  "IW{1,1}(12,:)'"/1 -> dotprod12/1
  dotprod12/1 -> Mux/12
  "IW{1,1}(13,:)'"/1 -> dotprod13/1
  dotprod13/1 -> Mux/13
  "IW{1,1}(14,:)'"/1 -> dotprod14/1
  dotprod14/1 -> Mux/14
  "IW{1,1}(15,:)'"/1 -> dotprod15/1
  dotprod15/1 -> Mux/15
  Mux/1 -> "iz{1,1}"/1

== system Q_learning_rotor_v3_min_M_imp/Environment/F3/Layer 2/Delays 1 ==
  "p{2}" : Inport  PortDimensions=15
      mask Display: e = 0.06;c1 = [120 230 180]/255;c2 = ([120 230 180]+0)/(256+128);c3 = ([120 230 180]+128)/(256+128);patch([0 1 1 0],[0 0 1 1],c1);patch([0 1 1 1-e 1-e 0+e],[0 0 1 1-e 0+e 0+e],c2);patch([0 0 1 1-e 0+e 0+e],[0 1 1 1-e 1-e 0+e],c3);plot([0 1 1 0 0],[0 0 1 1 0]);
  mux : Mux  Inputs=1
      mask Display: e = 0.06;c1 = [120 150 230]/255;c2 = ([120 150 230]+0)/383;c3 = ([120 150 230]+128)/383;patch([0 1 1 0],[0 0 1 1],c1);patch([0 1 1 1-e 1-e 0+e],[0 0 1 1-e 0+e 0+e],c2);patch([0 0 1 1-e 0+e 0+e],[0 1 1 1-e 1-e 0+e],c3);plot([0 1 1 0 0],[0 0 1 1 0]);disp('Mux')
  "pd{2,1}" : Outport
      mask Display: e = 0.06;c1 = [120 230 180]/255;c2 = ([120 230 180]+0)/(256+128);c3 = ([120 230 180]+128)/(256+128);patch([0 1 1 0],[0 0 1 1],c1);patch([0 1 1 1-e 1-e 0+e],[0 0 1 1-e 0+e 0+e],c2);patch([0 0 1 1-e 0+e 0+e],[0 1 1 1-e 1-e 0+e],c3);plot([0 1 1 0 0],[0 0 1 1 0]);
  wires:
  "p{2}"/1 -> mux/1
  mux/1 -> "pd{2,1}"/1

== system Q_learning_rotor_v3_min_M_imp/Environment/F3/Layer 2/LW{2,1} ==
  "ad{2,1}" : Inport  PortDimensions=15
      mask Display: e = 0.06;c1 = [120 230 180]/255;c2 = ([120 230 180]+0)/(256+128);c3 = ([120 230 180]+128)/(256+128);patch([0 1 1 0],[0 0 1 1],c1);patch([0 1 1 1-e 1-e 0+e],[0 0 1 1-e 0+e 0+e],c2);patch([0 0 1 1-e 0+e 0+e],[0 1 1 1-e 1-e 0+e],c3);plot([0 1 1 0 0],[0 0 1 1 0]);
  "IW{2,1}(1,:)'" : Constant  Value=[-3.617594306433918216470146944629959762096405029296875;4.02640558418821559172329216380603611469268798828125;-3.234515089768903006728351101628504693508148193359375;-1.4739495354445899533146757676149718463420867919921875;2.8710019130520691987840109504759311676025390625;0.1363723444796345052321129287520307116210460662841796875;-1.496996753744781916140027533401735126972198486328125;-4.67582619968248192066084811813198029994964599609375;-1.2046706811599718900396283061127178370952606201171875;-4.35845704992661797660957745392806828022003173828125;-2.28128825068953222654499768395908176898956298828125;5.3857038849677110192715190351009368896484375;2.5065702664579792013910264358855783939361572265625;-2.23875268234986268822694910340942442417144775390625;-1.1284468873998025895133423546212725341320037841796875]
      mask Display: e = 0.06;c1 = [120 150 230]/255;c2 = ([120 150 230]+0)/383;c3 = ([120 150 230]+128)/383;patch([0 1 1 0],[0 0 1 1],c1);patch([0 1 1 1-e 1-e 0+e],[0 0 1 1-e 0+e 0+e],c2);patch([0 0 1 1-e 0+e 0+e],[0 1 1 1-e 1-e 0+e],c3);plot([0 1 1 0 0],[0 0 1 1 0]);disp('weights');
  Mux : Mux  Inputs=1
      mask Display: e = 0.06;c1 = [120 150 230]/255;c2 = ([120 150 230]+0)/383;c3 = ([120 150 230]+128)/383;patch([0 1 1 0],[0 0 1 1],c1);patch([0 1 1 1-e 1-e 0+e],[0 0 1 1-e 0+e 0+e],c2);patch([0 0 1 1-e 0+e 0+e],[0 1 1 1-e 1-e 0+e],c3);plot([0 1 1 0 0],[0 0 1 1 0]);disp('Mux');
  dotprod1 : neural/Weight Functions/dotprod
  "lz{2,1}" : Outport
      mask Display: e = 0.06;c1 = [120 230 180]/255;c2 = ([120 230 180]+0)/(256+128);c3 = ([120 230 180]+128)/(256+128);patch([0 1 1 0],[0 0 1 1],c1);patch([0 1 1 1-e 1-e 0+e],[0 0 1 1-e 0+e 0+e],c2);patch([0 0 1 1-e 0+e 0+e],[0 1 1 1-e 1-e 0+e],c3);plot([0 1 1 0 0],[0 0 1 1 0]);
  wires:
  "IW{2,1}(1,:)'"/1 -> dotprod1/1
  "ad{2,1}"/1 -> dotprod1/2
  dotprod1/1 -> Mux/1
  Mux/1 -> "lz{2,1}"/1

== matlab function Q_learning_rotor_v3_min_M_imp/Subsystem1/MATLAB Function ==
  data: u1 input; y output; u2 input; u3 input; u4 input
function y = fcn(u1,u2,u3,u4)
if u1<u3 && u2>0.5
    y=u4+1;
else
    y=0;
end

end
